simulink model "teste_motor_v10"  (R2025b)
settings: Solver=VariableStepAuto  StartTime=0.0  StopTime=10  RelTol=1e-3
undefined symbols (not defined in the file): fdesignblkfcn, gcbh, Kad, Kre
libraries: nesl_utility x26, fl_lib x25, simulink x19, dsparch4 x3, sdl_lib x2, simulink_extras x2, dspfdesign x1
(part 1 of 3)
CloseFcn:
  | try, close(h1_sdl_single_cylinder_engine), end
  | clear h1_sdl_single_cylinder_engine
  | 
  | clear simlog_sdl_single_cylinder_engine
  | clear logsout_sdl_single_cylinder_engine
settings Model: PacingRate=0.089000  Creator=The MathWorks, Inc.  LastModifiedBy=vclau
settings SolverCC: MaxZcPerStep=1.0
settings DataIOCC: SaveFormat=Array  SaveOutput=off  DSMLogging=off  SaveTime=off  ReturnWorkspaceOutputs=off  SignalLoggingName=logsout_sdl_single_cylinder_engine
settings DebuggingCC: AlgebraicLoopMsg=none  MaxConsecutiveZCsMsg=warning
settings ModelReferenceCC: EnableRefExpFcnMdlSchedulingChecks=on
settings RTWCC: GPUComputeCapability=3.5  DLArmComputeVersion=19.05
settings SimscapeCC: SimscapeLogType=all  SimscapeLogSimulationStatistics=on  SimscapeLogName=simlog_sdl_single_cylinder_engine  SimscapeLogLimitData=off

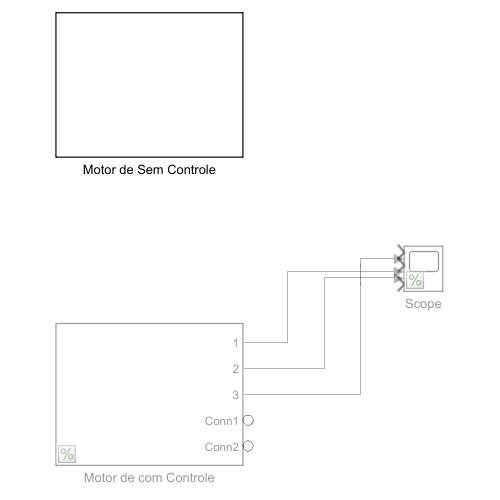
[thumbnail: Simulink's stored preview of the top-level diagram]
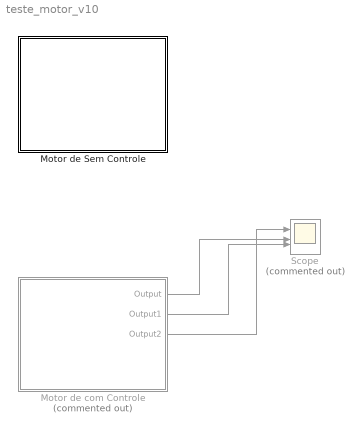
== system teste_motor_v10 ==
  Motor de Sem Controle : Subsystem
  Motor de com Controle : Subsystem  Commented=on
  Scope : Scope  Commented=on  NumInputPorts=6
      settings: ActiveDisplayYMinimum=-1  ActiveDisplayYMaximum=1
  wires:
  Motor de com Controle/1(Output) -> Scope/4
  Motor de com Controle/3(Output2) -> Scope/2
  Motor de com Controle/2(Output1) -> Scope/5

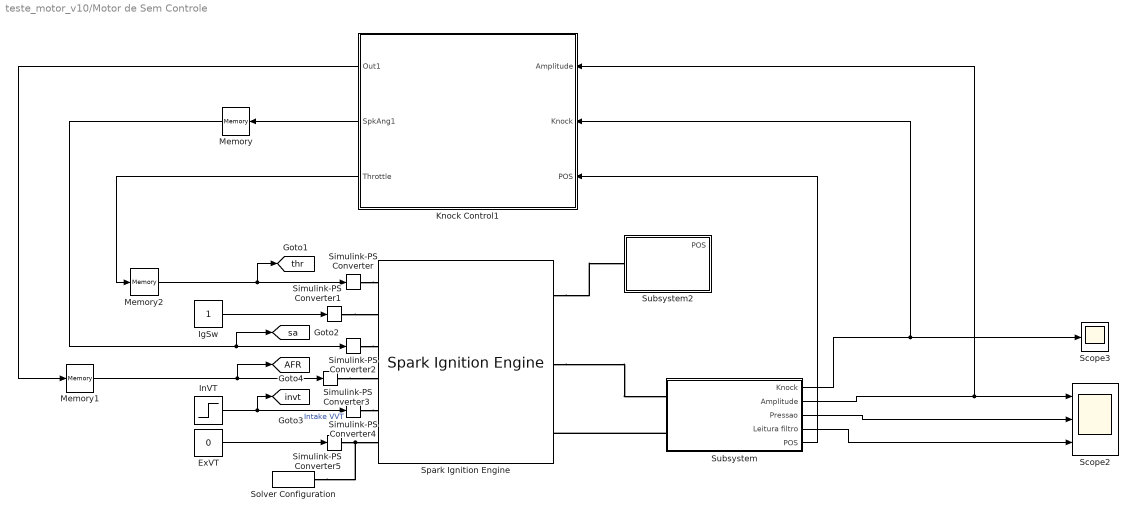
== system teste_motor_v10/Motor de Sem Controle ==
  ExVT : Constant  Value=0
  IgSw : Constant
  InVT : Step  Time=3  Before=30  After=0  SampleTime=0
  Knock Control1 : Subsystem
  Memory : Memory
  Memory1 : Memory  InitialCondition=14.7
  Memory2 : Memory
  Scope2 : Scope  NumInputPorts=3
      settings: ActiveDisplayYMinimum=-82.146412310849357  ActiveDisplayYMaximum=739.31771079764439  DataLoggingVariableName=ScopeData2
  Scope3 : Scope
      settings: ActiveDisplayYMinimum=0.61074348863970962  ActiveDisplayYMaximum=0.63050497432299946  DataLoggingVariableName=ScopeData3
  Simulink-PS Converter : nesl_utility/Simulink-PS Converter  PhysicalDomain=network_engine_domain  SubClassName=ps_input  LeftPortType=input  RightPortType=output  PseudoPeriodic=off  Frequencies=[]  NoiseDistribution=none  NoiseParameters=[]  Unit=1  AffineConversion=off  FilteringAndDerivatives=provide  SimscapeFilterOrder=1  InputFilterTimeConstant=0.001  UdotUserProvided=0
  Simulink-PS Converter1 : nesl_utility/Simulink-PS Converter  PhysicalDomain=network_engine_domain  SubClassName=ps_input  LeftPortType=input  RightPortType=output  PseudoPeriodic=off  Frequencies=[]  NoiseDistribution=none  NoiseParameters=[]  Unit=1  AffineConversion=off  FilteringAndDerivatives=provide  SimscapeFilterOrder=1  InputFilterTimeConstant=0.001  UdotUserProvided=0
  Simulink-PS Converter2 : nesl_utility/Simulink-PS Converter  PhysicalDomain=network_engine_domain  SubClassName=ps_input  LeftPortType=input  RightPortType=output  PseudoPeriodic=off  Frequencies=[]  NoiseDistribution=none  NoiseParameters=[]  Unit=deg  AffineConversion=off  FilteringAndDerivatives=provide  SimscapeFilterOrder=1  InputFilterTimeConstant=0.001  UdotUserProvided=0
  Simulink-PS Converter3 : nesl_utility/Simulink-PS Converter  PhysicalDomain=network_engine_domain  SubClassName=ps_input  LeftPortType=input  RightPortType=output  PseudoPeriodic=off  Frequencies=[]  NoiseDistribution=none  NoiseParameters=[]  Unit=1  AffineConversion=off  FilteringAndDerivatives=provide  SimscapeFilterOrder=1  InputFilterTimeConstant=0.001  UdotUserProvided=0
  Simulink-PS Converter4 : nesl_utility/Simulink-PS Converter  PhysicalDomain=network_engine_domain  SubClassName=ps_input  LeftPortType=input  RightPortType=output  PseudoPeriodic=off  Frequencies=[]  NoiseDistribution=none  NoiseParameters=[]  Unit=deg  AffineConversion=off  FilteringAndDerivatives=provide  SimscapeFilterOrder=1  InputFilterTimeConstant=0.001  UdotUserProvided=0
  Simulink-PS Converter5 : nesl_utility/Simulink-PS Converter  PhysicalDomain=network_engine_domain  SubClassName=ps_input  LeftPortType=input  RightPortType=output  PseudoPeriodic=off  Frequencies=[]  NoiseDistribution=none  NoiseParameters=[]  Unit=deg  AffineConversion=off  FilteringAndDerivatives=provide  SimscapeFilterOrder=1  InputFilterTimeConstant=0.001  UdotUserProvided=0
  Solver Configuration : nesl_utility/Solver Configuration  PhysicalDomain=network_engine_domain  SubClassName=solver  LeftPortType=input  RightPortType=generic  Tones=[]  Harmonics=[]  SimulateNoise=off  Profile=off  UseLocalSampling=off  EnableSwitchedLinearOptims=on  FrequencyDomain=off  UseCCode=off  RelTol=0.001  AbsTol=0.001  MinStep=1e-09  ToWorkspace=off  RevertToSquareIcSolve=off  NumHomotopyIterations=100  PhasorMode=off  PhasorModeNumHarmonics=1  ConsistencySolver=NEWTON_FTOL  IndexReductionMethod=DerivativeReplacement  DoDC=off  ResidualTolerance=1e-09  ConsistencyTolSource=GLOBAL  ConsistencyAbsTol=0.001  ConsistencyRelTol=0.001  ConsistencyTolFactor=0.001  UseLocalSolver=off  LocalSolverChoice=NE_BACKWARD_EULER_ADVANCER  ResolveIndetEquations=on  FunctionEvalNumThread=1  LocalSolverSampleTime=0.001  DoFixedCost=off  MaxNonlinIter=3  MaxModeIter=2  ComputeImpulses=off  ImpulseIterations=2  LinearAlgebra=auto  LinearAlgebraNumThread=0  EquationFormulation=NE_TIME_EF  DelaysMemoryBudget=1024  AutomaticFiltering=on  FilteringTimeConstant=0.001  PartitionStorageMethod=AS_NEEDED  PartitionMemoryBudget=1024  PartitionMethod=ROBUST  MultibodyUseLocalSolver=off  MultibodyLocalSolverChoice=ODE1  MultibodyLocalSolverSampleTime=0.001
  Spark Ignition Engine : sdl_lib/Engines & Motors/Spark Ignition Engine  numCyls=sdl.enum.engineNumCylinders.One  twoCylSADiff=270 deg  L4FiringOrder=sdl.enum.engineFiringOrderFourCylinders.L4_1342  bore=72 mm  stroke=61 mm  conrod=97 mm  CR=11.3  P_amb=101.325 kPa  T_amb=298.15 K  rho_air=1.225 mg/cm^3  R_air=288.1965 J/(K*kg)  UseAirIntake=simscape.enum.onoff.on  c_thr=0.05 s  thr_rest=3 deg  D_plate=5 cm  S_leak=1 cm^2  V_im=500 cm^3  Cd_in=0.9  IVO_0=5 deg  IVC_0=60 deg  EVO_0=60 deg  EVC_0=5 deg  UseInVVT=simscape.enum.onoff.on  UseExVVT=simscape.enum.onoff.on  q_LHV=44.3 MJ/kg  InputAFR=simscape.enum.onoff.on  AFR_const=14.6  InputInjPw=simscape.enum.onoff.off  Sinj=6.5 mg/ms  SparkInputType=sdl.enum.engineSparkInputType.Angle  SA_const=20 deg  comb_bd=50 deg  dt_Pcyl_slow_decay=60 s  dt_Tcyl_slow_decay=600 s  dt_exh_decay=5 ms  InputBackPressure=simscape.enum.onoff.off  dP_exh=50 kPa  dw_exh=6000 rpm  UseExhaustThermal=simscape.enum.onoff.on  S_exh=1 m^2  M_exh=5 kg  C_exh=100 J/(K*kg)  k_gas=10 s  h_convection=100 W/(K*m^2)  k_radiation=0.3  SB=5.7e-8 W/(K^4*m^2)  Pim_0=101.325 kPa  ca0=0 deg  w0=1000 rpm  EngSpdSimLimit=10000 rpm  OutputTorqueAvr=simscape.enum.onoff.off  OutputSpeedAvr=simscape.enum.onoff.off  OutputCrkpos=simscape.enum.onoff.on  OutputPim=simscape.enum.onoff.off  OutputAirMassFlow=simscape.enum.onoff.off  OutputFuelMassFlow=simscape.enum.onoff.off  OutputAFR=false  OutputVcyl=false  OutputPcyl=simscape.enum.onoff.on  OutputTcyl=simscape.enum.onoff.off  OutputTexh=simscape.enum.onoff.off
      settings: AttributesFormatString=%<w0> [%<w0_unit>]  InternalSimscapePortConfiguration="{\"Bottom\":[],\"Left\":[{\"id\":\"thr_cmd\",\"label\":\"Thr\",\"type\":\"input\"},{\"id\":\"IGSW\",\"label\":\"IgSw\",\"type\":\"input\"},{\"id\":\"sa\",\"label\":\"SA\",\"type\":\"input\"},{\"id\":\"afr_in\",\"label\":\"AfrCmd\",\"type\":\"input\"},{\"id\":\"dIV\",\"label\":\"InVT\",\"type\":\"input\"},{\"id\":\"dEV\",\"label\":\"ExVT\",\"type\":\"input\"}],\"Right\":[{\"id\":\"F\",\"label\":\"F\",\"type\":\"foundation.mechanical.rotational.rotational\"},{\"id\":\"crkpos\",\"label\":\"crkpos\",\"type\":\"output\"},{\"id\":\"P_out\",\"label\":\"Pcyl\",\"type\":\"output\"}],\"Top\":[]}"
  Subsystem : Subsystem
  Subsystem2 : Subsystem
  tag scope: AFR=global, invt=global, sa=global, thr=global
  wires:
  IgSw/1 -> Simulink-PS Converter1/1
  ExVT/1 -> Simulink-PS Converter5/1
  InVT/1 -> [invt], Simulink-PS Converter4/1  "Intake VVT"
  Subsystem/1(Knock) -> Knock Control1/2(Knock), Scope3/1
  Subsystem/2(Amplitude) -> Knock Control1/1(Amplitude), Scope2/1
  Subsystem/3(Pressao) -> Scope2/2
  Subsystem/4(Leitura filtro) -> Scope2/3
  Subsystem/5(POS) -> Knock Control1/3(POS)
  Memory/1 -> [sa], Simulink-PS Converter2/1
  Knock Control1/1(Out1) -> Memory1/1
  Memory1/1 -> [AFR], Simulink-PS Converter3/1
  Knock Control1/2(SpkAng1) -> Memory/1
  Knock Control1/3(Throttle) -> Memory2/1
  Memory2/1 -> [thr], Simulink-PS Converter/1
  connections:
  Simulink-PS Converter1/RConn1 -- Spark Ignition Engine/LConn2
  Simulink-PS Converter4/RConn1 -- Spark Ignition Engine/LConn5
  Simulink-PS Converter3/RConn1 -- Spark Ignition Engine/LConn4
  Simulink-PS Converter2/RConn1 -- Spark Ignition Engine/LConn3
  Simulink-PS Converter/RConn1 -- Spark Ignition Engine/LConn1
  Simulink-PS Converter5/RConn1 -- Solver Configuration/RConn1 -- Spark Ignition Engine/LConn6
  Spark Ignition Engine/RConn2 -- Subsystem/LConn1
  Subsystem/LConn2 -- Spark Ignition Engine/RConn3
  Spark Ignition Engine/RConn1 -- Subsystem2/LConn1

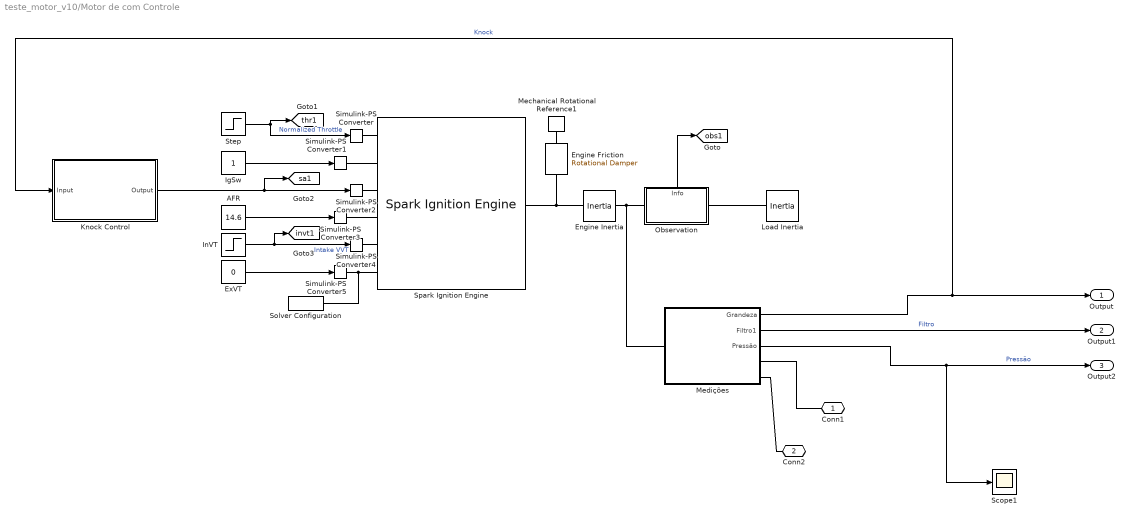
== system teste_motor_v10/Motor de com Controle ==
  AFR : Constant  Value=14.6
  Engine Friction : fl_lib/Mechanical/Rotational Elements/Rotational Damper  D=0.01 N*m/rpm  w_specify=off  w_priority=None  w=0 rad/s  w_nominal_specify=off  w_nominal_value=1  w_nominal_unit=rad/s  t_specify=off  t_priority=None  t=0 N*m  t_nominal_specify=off  t_nominal_value=1  t_nominal_unit=N*m
      settings: AttributesFormatString=%<D> [%<D_unit>]
  Engine Inertia : fl_lib/Mechanical/Rotational Elements/Inertia  inertia=0.01 kg*m^2  num_ports=foundation.enum.numPorts2.two  w_specify=on  w_priority=High  w=1000 rpm  w_nominal_specify=off  w_nominal_value=1  w_nominal_unit=rad/s  t_specify=off  t_priority=None  t=0 N*m  t_nominal_specify=off  t_nominal_value=1  t_nominal_unit=N*m
      settings: InternalSimscapePortConfiguration="{\"Bottom\":[],\"Left\":[{\"id\":\"I\",\"label\":\"\",\"type\":\"foundation.mechanical.rotational.rotational\"}],\"Right\":[{\"id\":\"J\",\"label\":\"\",\"type\":\"foundation.mechanical.rotational.rotational\"}],\"Top\":[]}"
      settings: AttributesFormatString=|
      | Initial: %<w> [%<w_unit>]
      | %<inertia> [%<inertia_unit>]
  ExVT : Constant  Value=0
  IgSw : Constant
  InVT : Step  Time=3  Before=30  After=0  SampleTime=0
  Knock Control : Subsystem
  Load Inertia : fl_lib/Mechanical/Rotational Elements/Inertia  inertia=10*0.1^2 kg*m^2  num_ports=foundation.enum.numPorts2.one  w_specify=on  w_priority=None  w=0 rpm  w_nominal_specify=off  w_nominal_value=1  w_nominal_unit=rad/s  t_specify=off  t_priority=None  t=0 N*m  t_nominal_specify=off  t_nominal_value=1  t_nominal_unit=N*m
      settings: AttributesFormatString=|
      | Initial: %<w> [%<w_unit>]
      | %<inertia> [%<inertia_unit>]
  Mechanical Rotational Reference1 : fl_lib/Mechanical/Rotational Elements/Mechanical Rotational Reference
  Medições : Subsystem
  Observation : Subsystem
      settings: PortSchema="{\"entries\":[{\"content\":{\"sides\":[{\"content\":{\"connectorIds\":[\"LConn1\"]},\"type\":\"ConnectorPlacement.EquallySpacedRectSide\",\"uuid\":\"410be9a6-c4e5-432d-8066-24e0f4965a53\"},{\"content\":{\"connectorIds\":[\"RConn1\"],\"side\":\"RIGHT\"},\"type\":\"ConnectorPlacement.EquallySpacedRectSide\",\"uuid\":\"7b59f0c0-a218-4635-982c-3ab19ae33344\"},{\"content\":{\"connectorIds\":[\"Out1\"],\"side\":\"TOP\"},\"type\":\"ConnectorPlacement.EquallySpacedRectSide\",\"uuid\":\"569b4327-99bc-47a9-a8b7-c1caa6dee46d\"}]},\"type\":\"ConnectorPlacement.EquallySpacedConnector\",\"uuid\":\"611a8619-a64a-4be7-a61a-aa8fabb87e61\"}],\"packageUris\":[\"http://schema.mathworks.com/mf0/Connector/R2020b\"],\"version\":\"1.0\"}"
  Scope1 : Scope
      settings: ActiveDisplayYMinimum=101298.89151  ActiveDisplayYMaximum=101559.9764  DataLoggingVariableName=ScopeData3
  Simulink-PS Converter : nesl_utility/Simulink-PS Converter  PhysicalDomain=network_engine_domain  SubClassName=ps_input  LeftPortType=input  RightPortType=output  PseudoPeriodic=off  Frequencies=[]  NoiseDistribution=none  NoiseParameters=[]  Unit=1  AffineConversion=off  FilteringAndDerivatives=provide  SimscapeFilterOrder=1  InputFilterTimeConstant=0.001  UdotUserProvided=0
  Simulink-PS Converter1 : nesl_utility/Simulink-PS Converter  PhysicalDomain=network_engine_domain  SubClassName=ps_input  LeftPortType=input  RightPortType=output  PseudoPeriodic=off  Frequencies=[]  NoiseDistribution=none  NoiseParameters=[]  Unit=1  AffineConversion=off  FilteringAndDerivatives=provide  SimscapeFilterOrder=1  InputFilterTimeConstant=0.001  UdotUserProvided=0
  Simulink-PS Converter2 : nesl_utility/Simulink-PS Converter  PhysicalDomain=network_engine_domain  SubClassName=ps_input  LeftPortType=input  RightPortType=output  PseudoPeriodic=off  Frequencies=[]  NoiseDistribution=none  NoiseParameters=[]  Unit=deg  AffineConversion=off  FilteringAndDerivatives=provide  SimscapeFilterOrder=1  InputFilterTimeConstant=0.001  UdotUserProvided=0
  Simulink-PS Converter3 : nesl_utility/Simulink-PS Converter  PhysicalDomain=network_engine_domain  SubClassName=ps_input  LeftPortType=input  RightPortType=output  PseudoPeriodic=off  Frequencies=[]  NoiseDistribution=none  NoiseParameters=[]  Unit=1  AffineConversion=off  FilteringAndDerivatives=provide  SimscapeFilterOrder=1  InputFilterTimeConstant=0.001  UdotUserProvided=0
  Simulink-PS Converter4 : nesl_utility/Simulink-PS Converter  PhysicalDomain=network_engine_domain  SubClassName=ps_input  LeftPortType=input  RightPortType=output  PseudoPeriodic=off  Frequencies=[]  NoiseDistribution=none  NoiseParameters=[]  Unit=deg  AffineConversion=off  FilteringAndDerivatives=provide  SimscapeFilterOrder=1  InputFilterTimeConstant=0.001  UdotUserProvided=0
  Simulink-PS Converter5 : nesl_utility/Simulink-PS Converter  PhysicalDomain=network_engine_domain  SubClassName=ps_input  LeftPortType=input  RightPortType=output  PseudoPeriodic=off  Frequencies=[]  NoiseDistribution=none  NoiseParameters=[]  Unit=deg  AffineConversion=off  FilteringAndDerivatives=provide  SimscapeFilterOrder=1  InputFilterTimeConstant=0.001  UdotUserProvided=0
  Solver Configuration : nesl_utility/Solver Configuration  PhysicalDomain=network_engine_domain  SubClassName=solver  LeftPortType=input  RightPortType=generic  Tones=[]  Harmonics=[]  SimulateNoise=off  Profile=off  UseLocalSampling=off  EnableSwitchedLinearOptims=on  FrequencyDomain=off  UseCCode=off  RelTol=0.001  AbsTol=0.001  MinStep=1e-09  ToWorkspace=off  RevertToSquareIcSolve=off  NumHomotopyIterations=100  PhasorMode=off  PhasorModeNumHarmonics=1  ConsistencySolver=NEWTON_FTOL  IndexReductionMethod=DerivativeReplacement  DoDC=off  ResidualTolerance=1e-09  ConsistencyTolSource=GLOBAL  ConsistencyAbsTol=0.001  ConsistencyRelTol=0.001  ConsistencyTolFactor=0.001  UseLocalSolver=off  LocalSolverChoice=NE_BACKWARD_EULER_ADVANCER  ResolveIndetEquations=on  FunctionEvalNumThread=1  LocalSolverSampleTime=0.001  DoFixedCost=off  MaxNonlinIter=3  MaxModeIter=2  ComputeImpulses=off  ImpulseIterations=2  LinearAlgebra=auto  LinearAlgebraNumThread=0  EquationFormulation=NE_TIME_EF  DelaysMemoryBudget=1024  AutomaticFiltering=on  FilteringTimeConstant=0.001  PartitionStorageMethod=AS_NEEDED  PartitionMemoryBudget=1024  PartitionMethod=ROBUST  MultibodyUseLocalSolver=off  MultibodyLocalSolverChoice=ODE1  MultibodyLocalSolverSampleTime=0.001
  Spark Ignition Engine : sdl_lib/Engines & Motors/Spark Ignition Engine  numCyls=sdl.enum.engineNumCylinders.One  twoCylSADiff=270 deg  L4FiringOrder=sdl.enum.engineFiringOrderFourCylinders.L4_1342  bore=72 mm  stroke=61 mm  conrod=97 mm  CR=11.3  P_amb=101.325 kPa  T_amb=298.15 K  rho_air=1.225 mg/cm^3  R_air=288.1965 J/(K*kg)  UseAirIntake=simscape.enum.onoff.on  c_thr=0.05 s  thr_rest=3 deg  D_plate=5 cm  S_leak=1 cm^2  V_im=500 cm^3  Cd_in=0.9  IVO_0=5 deg  IVC_0=60 deg  EVO_0=60 deg  EVC_0=5 deg  UseInVVT=simscape.enum.onoff.on  UseExVVT=simscape.enum.onoff.on  q_LHV=44.3 MJ/kg  InputAFR=simscape.enum.onoff.on  AFR_const=14.6  InputInjPw=simscape.enum.onoff.off  Sinj=6.5 mg/ms  SparkInputType=sdl.enum.engineSparkInputType.Angle  SA_const=20 deg  comb_bd=50 deg  dt_Pcyl_slow_decay=60 s  dt_Tcyl_slow_decay=600 s  dt_exh_decay=5 ms  InputBackPressure=simscape.enum.onoff.off  dP_exh=50 kPa  dw_exh=6000 rpm  UseExhaustThermal=simscape.enum.onoff.on  S_exh=1 m^2  M_exh=5 kg  C_exh=100 J/(K*kg)  k_gas=10 s  h_convection=100 W/(K*m^2)  k_radiation=0.3  SB=5.7e-8 W/(K^4*m^2)  Pim_0=101.325 kPa  ca0=0 deg  w0=1000 rpm  EngSpdSimLimit=10000 rpm  OutputTorqueAvr=simscape.enum.onoff.off  OutputSpeedAvr=simscape.enum.onoff.off  OutputCrkpos=simscape.enum.onoff.off  OutputPim=simscape.enum.onoff.off  OutputAirMassFlow=simscape.enum.onoff.off  OutputFuelMassFlow=simscape.enum.onoff.off  OutputAFR=simscape.enum.onoff.off  OutputVcyl=simscape.enum.onoff.off  OutputPcyl=simscape.enum.onoff.off  OutputTcyl=simscape.enum.onoff.off  OutputTexh=simscape.enum.onoff.off
      settings: AttributesFormatString=%<w0> [%<w0_unit>]  InternalSimscapePortConfiguration="{\"Bottom\":[],\"Left\":[{\"id\":\"thr_cmd\",\"label\":\"Thr\",\"type\":\"input\"},{\"id\":\"IGSW\",\"label\":\"IgSw\",\"type\":\"input\"},{\"id\":\"sa\",\"label\":\"SA\",\"type\":\"input\"},{\"id\":\"afr_in\",\"label\":\"AfrCmd\",\"type\":\"input\"},{\"id\":\"dIV\",\"label\":\"InVT\",\"type\":\"input\"},{\"id\":\"dEV\",\"label\":\"ExVT\",\"type\":\"input\"}],\"Right\":[{\"id\":\"F\",\"label\":\"F\",\"type\":\"foundation.mechanical.rotational.rotational\"}],\"Top\":[]}"
  Step : Step  Time=15  Before=0.2  SampleTime=0
  Conn1 : PMIOPort  Side=Right
  Conn2 : PMIOPort  Port=2  Side=Right
  Output : Outport
  Output1 : Outport  Port=2
  Output2 : Outport  Port=3
  tag scope: invt1=global, obs1=global, sa1=global, thr1=global
  wires:
  IgSw/1 -> Simulink-PS Converter1/1
  Medições/2(Filtro1) -> Output1/1  "Filtro"
  AFR/1 -> Simulink-PS Converter3/1
  Step/1 -> Simulink-PS Converter/1, [thr1]  "Normalized Throttle"
  Observation/1(Info) -> [obs1]
  Medições/1(Grandeza) -> Output/1, Knock Control/1(Input)  "Knock"
  Knock Control/1(Output) -> [sa1], Simulink-PS Converter2/1
  ExVT/1 -> Simulink-PS Converter5/1
  Medições/3(Pressão) -> Output2/1, Scope1/1  "Pressão"
  InVT/1 -> [invt1], Simulink-PS Converter4/1  "Intake VVT"
  connections:
  Medições/RConn1 -- Conn1/RConn1
  Spark Ignition Engine/RConn1 -- Engine Friction/LConn1 -- Engine Inertia/RConn1
  Simulink-PS Converter1/RConn1 -- Spark Ignition Engine/LConn2
  Mechanical Rotational Reference1/LConn1 -- Engine Friction/RConn1
  Simulink-PS Converter4/RConn1 -- Spark Ignition Engine/LConn5
  Observation/RConn1 -- Load Inertia/LConn1
  Simulink-PS Converter3/RConn1 -- Spark Ignition Engine/LConn4
  Simulink-PS Converter2/RConn1 -- Spark Ignition Engine/LConn3
  Simulink-PS Converter/RConn1 -- Spark Ignition Engine/LConn1
  Engine Inertia/LConn1 -- Medições/LConn1 -- Observation/LConn1
  Simulink-PS Converter5/RConn1 -- Solver Configuration/RConn1 -- Spark Ignition Engine/LConn6
  Medições/RConn2 -- Conn2/RConn1

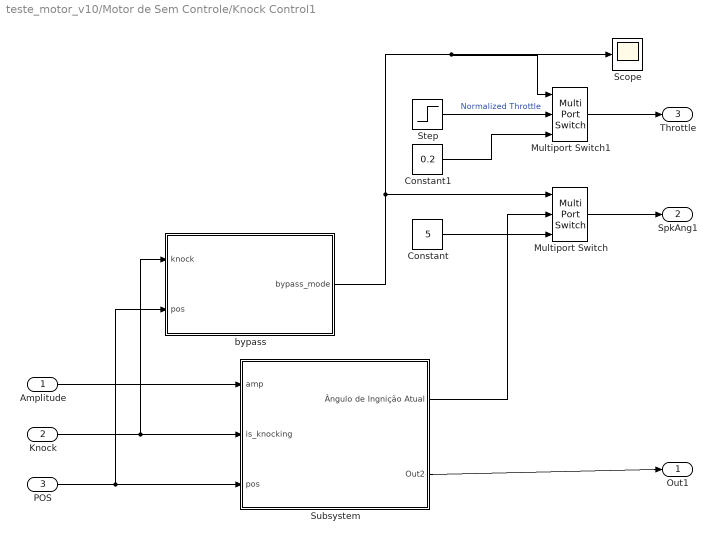
== system teste_motor_v10/Motor de Sem Controle/Knock Control1 ==
  Amplitude : Inport
  Knock : Inport  Port=2
  POS : Inport  Port=3
  Constant : Constant  Value=5
  Constant1 : Constant  Value=0.2
  Multiport Switch : MultiPortSwitch  Inputs=2  SaturateOnIntegerOverflow=off  InputSameDT=off
  Multiport Switch1 : MultiPortSwitch  Inputs=2  SaturateOnIntegerOverflow=off  InputSameDT=off
  Scope : Scope
      settings: ActiveDisplayYMinimum=0.875  ActiveDisplayYMaximum=2.125  DataLoggingVariableName=ScopeData12
  Step : Step  Before=0.2  SampleTime=0
  Subsystem : Subsystem
  bypass : MATLAB Function  TreatAsAtomicUnit=on
  Out1 : Outport
  SpkAng1 : Outport  Port=2
  Throttle : Outport  Port=3
  wires:
  Amplitude/1 -> Subsystem/1(amp)
  Knock/1 -> bypass/1(knock), Subsystem/2(is_knocking)
  POS/1 -> bypass/2(pos), Subsystem/3(pos)
  Subsystem/2(Out2) -> Out1/1
  Subsystem/1(Ângulo de Ingnição Atual) -> Multiport Switch/2
  Multiport Switch/1 -> SpkAng1/1
  Multiport Switch1/1 -> Throttle/1
  Step/1 -> Multiport Switch1/2  "Normalized Throttle"
  bypass/1(bypass_mode) -> Scope/1, Multiport Switch1/1, Multiport Switch/1
  Constant/1 -> Multiport Switch/3
  Constant1/1 -> Multiport Switch1/3

== system teste_motor_v10/Motor de Sem Controle/Subsystem ==
  Filtro : Subsystem
  Leituras : Subsystem
  Threshold e Sensor : Subsystem
  Crank Angle : PMIOPort  Side=Left
  Pressão : PMIOPort  Port=2  Side=Left
  Knock : Outport
  Amplitude : Outport  Port=2
  Pressao : Outport  Port=3
  Leitura filtro : Outport  Port=4
  POS : Outport  Port=5
  wires:
  Leituras/1(Pressão com Knock) -> Pressao/1, Filtro/1(Pressão com Knock)
  Threshold e Sensor/1(Knock) -> Knock/1
  Filtro/2(Filtro) -> Leitura filtro/1
  Threshold e Sensor/2(Amplitude) -> Amplitude/1
  Filtro/1(Sinal filtrado) -> Threshold e Sensor/1(Sinal filtrado)
  Leituras/2(CrkAng) -> POS/1
  connections:
  Crank Angle/RConn1 -- Leituras/LConn1
  Leituras/LConn2 -- Pressão/RConn1

== system teste_motor_v10/Motor de Sem Controle/Subsystem2 ==
  Engine Friction : fl_lib/Mechanical/Rotational Elements/Rotational Damper  D=0.01 N*m/rpm  w_specify=off  w_priority=None  w=0 rad/s  w_nominal_specify=off  w_nominal_value=1  w_nominal_unit=rad/s  t_specify=off  t_priority=None  t=0 N*m  t_nominal_specify=off  t_nominal_value=1  t_nominal_unit=N*m
      settings: AttributesFormatString=%<D> [%<D_unit>]
  Engine Inertia : fl_lib/Mechanical/Rotational Elements/Inertia  inertia=0.01 kg*m^2  num_ports=foundation.enum.numPorts2.two  w_specify=on  w_priority=High  w=1000 rpm  w_nominal_specify=off  w_nominal_value=1  w_nominal_unit=rad/s  t_specify=off  t_priority=None  t=0 N*m  t_nominal_specify=off  t_nominal_value=1  t_nominal_unit=N*m
      settings: InternalSimscapePortConfiguration="{\"Bottom\":[],\"Left\":[{\"id\":\"I\",\"label\":\"\",\"type\":\"foundation.mechanical.rotational.rotational\"}],\"Right\":[{\"id\":\"J\",\"label\":\"\",\"type\":\"foundation.mechanical.rotational.rotational\"}],\"Top\":[]}"
      settings: AttributesFormatString=|
      | Initial: %<w> [%<w_unit>]
      | %<inertia> [%<inertia_unit>]
  Load Inertia : fl_lib/Mechanical/Rotational Elements/Inertia  inertia=10*0.1^2 kg*m^2  num_ports=foundation.enum.numPorts2.one  w_specify=on  w_priority=None  w=0 rpm  w_nominal_specify=off  w_nominal_value=1  w_nominal_unit=rad/s  t_specify=off  t_priority=None  t=0 N*m  t_nominal_specify=off  t_nominal_value=1  t_nominal_unit=N*m
      settings: AttributesFormatString=|
      | Initial: %<w> [%<w_unit>]
      | %<inertia> [%<inertia_unit>]
  Mechanical Rotational Reference1 : fl_lib/Mechanical/Rotational Elements/Mechanical Rotational Reference
  Observation : Subsystem
      settings: PortSchema="{\"entries\":[{\"content\":{\"sides\":[{\"content\":{\"connectorIds\":[\"LConn1\"]},\"type\":\"ConnectorPlacement.EquallySpacedRectSide\",\"uuid\":\"410be9a6-c4e5-432d-8066-24e0f4965a53\"},{\"content\":{\"connectorIds\":[\"RConn1\"],\"side\":\"RIGHT\"},\"type\":\"ConnectorPlacement.EquallySpacedRectSide\",\"uuid\":\"7b59f0c0-a218-4635-982c-3ab19ae33344\"},{\"content\":{\"connectorIds\":[\"Out1\"],\"side\":\"TOP\"},\"type\":\"ConnectorPlacement.EquallySpacedRectSide\",\"uuid\":\"569b4327-99bc-47a9-a8b7-c1caa6dee46d\"}]},\"type\":\"ConnectorPlacement.EquallySpacedConnector\",\"uuid\":\"611a8619-a64a-4be7-a61a-aa8fabb87e61\"}],\"packageUris\":[\"http://schema.mathworks.com/mf0/Connector/R2020b\"],\"version\":\"1.0\"}"
  Subsystem1 : Subsystem
  Conn1 : PMIOPort  Side=Left
  Conn2 : PMIOPort  Port=2  Side=Right
  Conn3 : PMIOPort  Port=3  Side=Right
  POS : Outport
  tag scope: obs=global
  wires:
  Subsystem1/1(POS) -> POS/1
  Observation/1(Info) -> [obs]
  connections:
  Engine Friction/LConn1 -- Conn1/RConn1 -- Engine Inertia/RConn1
  Mechanical Rotational Reference1/LConn1 -- Engine Friction/RConn1
  Engine Inertia/LConn1 -- Subsystem1/LConn1 -- Observation/LConn1
  Subsystem1/RConn1 -- Conn2/RConn1
  Observation/RConn1 -- Load Inertia/LConn1
  Subsystem1/RConn2 -- Conn3/RConn1

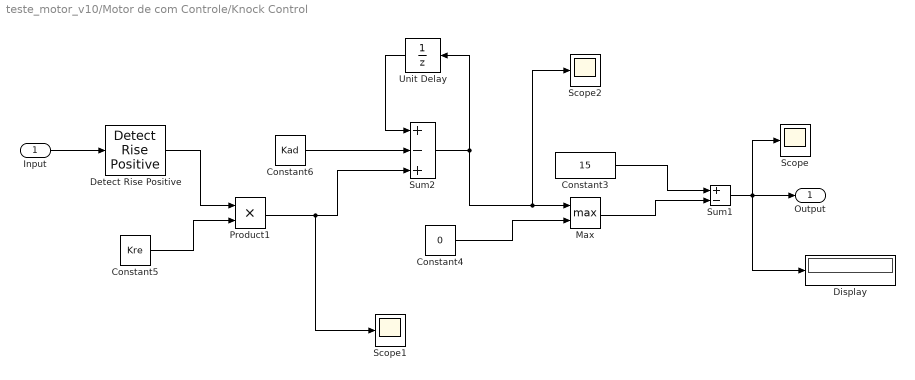
== system teste_motor_v10/Motor de com Controle/Knock Control ==
  Input : Inport
  Constant3 : Constant  Value=15
  Constant4 : Constant  Value=0
  Constant5 : Constant  Value=Kre
  Constant6 : Constant  Value=Kad
  Detect Rise Positive : simulink/Logic and Bit Operations/Detect Rise Positive  vinit=0  OutDataTypeStr=boolean
  Display : Display
  Max : MinMax  Function=max  Inputs=2
  Product1 : Product
  Scope : Scope
      settings: ActiveDisplayYMinimum=11.265  ActiveDisplayYMaximum=15.415
  Scope1 : Scope
      settings: ActiveDisplayYMinimum=-0.625  ActiveDisplayYMaximum=5.625
  Scope2 : Scope
      settings: ActiveDisplayYMinimum=-23.7475  ActiveDisplayYMaximum=6.3275  DataLoggingVariableName=ScopeData2
  Sum1 : Sum  Inputs=+-
  Sum2 : Sum  Inputs=+-+
  Unit Delay : UnitDelay  SampleTime=-1  HasFrameUpgradeWarning=on
  Output : Outport
  wires:
  Constant3/1 -> Sum1/1
  Max/1 -> Sum1/2
  Sum2/1 -> Unit Delay/1, Scope2/1, Max/1
  Product1/1 -> Scope1/1, Sum2/3
  Constant4/1 -> Max/2
  Constant6/1 -> Sum2/2
  Constant5/1 -> Product1/2
  Sum1/1 -> Display/1, Scope/1, Output/1
  Unit Delay/1 -> Sum2/1
  Detect Rise Positive/1 -> Product1/1
  Input/1 -> Detect Rise Positive/1

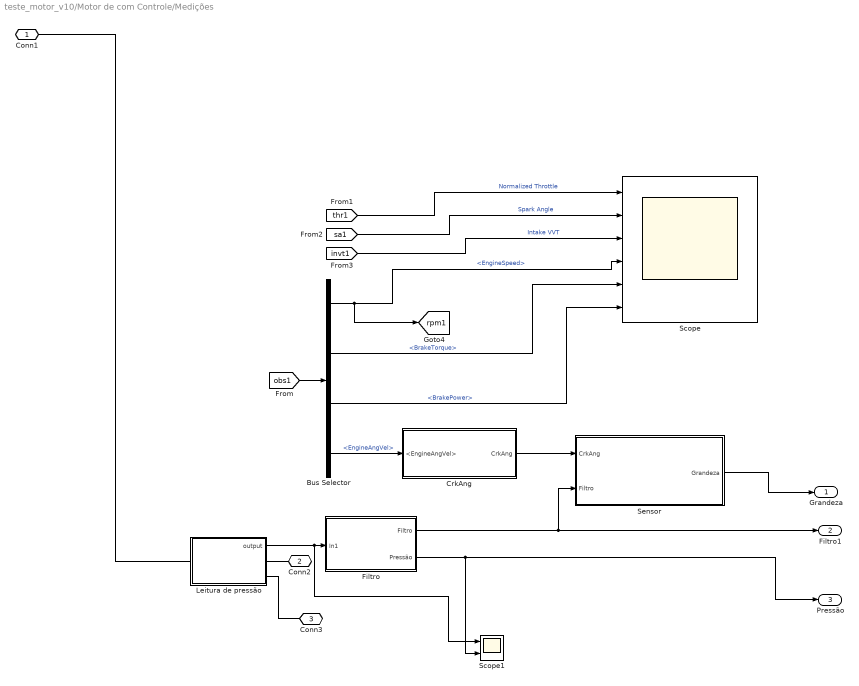
== system teste_motor_v10/Motor de com Controle/Medições ==
  Bus Selector : BusSelector  OutputSignals=EngineSpeed,BrakeTorque,BrakePower,EngineAngVel
  CrkAng : Subsystem
  Filtro : Subsystem
  Leitura de pressão : Subsystem
  Scope : Scope  NumInputPorts=6
      settings: ActiveDisplayYMinimum=0.1  ActiveDisplayYMaximum=1.1
  Scope1 : Scope  NumInputPorts=2
      settings: ActiveDisplayYMinimum=94814.33534  ActiveDisplayYMaximum=119364.22182  DataLoggingVariableName=ScopeData5
  Sensor : Subsystem
  Conn1 : PMIOPort  Side=Left
  Conn2 : PMIOPort  Port=2  Side=Right
  Conn3 : PMIOPort  Port=3  Side=Right
  Grandeza : Outport
  Filtro1 : Outport  Port=2
  Pressão : Outport  Port=3
  tag scope: rpm1=global
  wires:
  [invt1] -> Scope/3  "Intake VVT"
  CrkAng/1(CrkAng) -> Sensor/1(CrkAng)
  Filtro/1(Filtro) -> Filtro1/1, Sensor/2(Filtro)
  [obs1] -> Bus Selector/1
  Bus Selector/4 -> CrkAng/1(<EngineAngVel>)  "<EngineAngVel>"
  Leitura de pressão/1(output) -> Scope1/1, Filtro/1(In1)
  Bus Selector/2 -> Scope/5  "<BrakeTorque>"
  Bus Selector/3 -> Scope/6  "<BrakePower>"
  Bus Selector/1 -> [rpm1], Scope/4  "<EngineSpeed>"
  [sa1] -> Scope/2  "Spark Angle"
  [thr1] -> Scope/1  "Normalized Throttle"
  Filtro/2(Pressão) -> Scope1/2, Pressão/1
  Sensor/1(Grandeza) -> Grandeza/1
  connections:
  Leitura de pressão/RConn1 -- Conn2/RConn1
  Leitura de pressão/LConn1 -- Conn1/RConn1
  Leitura de pressão/RConn2 -- Conn3/RConn1

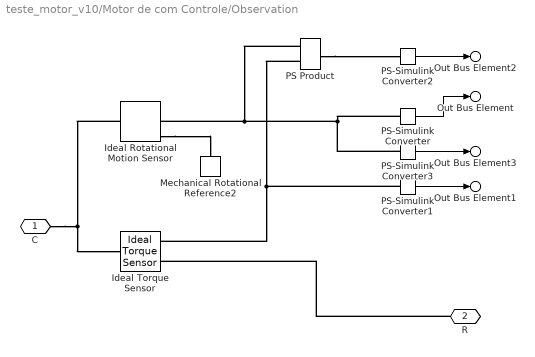
== system teste_motor_v10/Motor de com Controle/Observation ==
  Ideal Rotational Motion Sensor : fl_lib/Mechanical/Mechanical Sensors/Ideal Rotational Motion Sensor  reference=foundation.enum.MeasurementReference.difference  acceleration_port=false  velocity_port=true  position_port=true  wrap_angle=simscape.enum.onoff.off  offset=0 rad
  Ideal Torque Sensor : fl_lib/Mechanical/Mechanical Sensors/Ideal Torque Sensor
  Mechanical Rotational Reference2 : fl_lib/Mechanical/Rotational Elements/Mechanical Rotational Reference
  PS Product : fl_lib/Physical Signals/Functions/PS Product
  PS-Simulink Converter : nesl_utility/PS-Simulink Converter  PhysicalDomain=network_engine_domain  SubClassName=ps_output  LeftPortType=input  RightPortType=output  PseudoPeriodic=off  Frequencies=[]  VectorFormat=inherit  Unit=rpm  AffineConversion=off
  PS-Simulink Converter1 : nesl_utility/PS-Simulink Converter  PhysicalDomain=network_engine_domain  SubClassName=ps_output  LeftPortType=input  RightPortType=output  PseudoPeriodic=off  Frequencies=[]  VectorFormat=inherit  Unit=N*m  AffineConversion=off
  PS-Simulink Converter2 : nesl_utility/PS-Simulink Converter  PhysicalDomain=network_engine_domain  SubClassName=ps_output  LeftPortType=input  RightPortType=output  PseudoPeriodic=off  Frequencies=[]  VectorFormat=inherit  Unit=kW  AffineConversion=off
  PS-Simulink Converter3 : nesl_utility/PS-Simulink Converter  PhysicalDomain=network_engine_domain  SubClassName=ps_output  LeftPortType=input  RightPortType=output  PseudoPeriodic=off  Frequencies=[]  VectorFormat=inherit  Unit=rad/s  AffineConversion=off
  C : PMIOPort  Side=Left
  R : PMIOPort  Port=2  Side=Right
  Out Bus Element : Outport  PortName=Info  Element=EngineSpeed
      settings: AttributesFormatString=%<Unit>
  Out Bus Element1 : Outport  PortName=Info  Element=BrakeTorque
      settings: AttributesFormatString=%<Unit>
  Out Bus Element2 : Outport  PortName=Info  Element=BrakePower
      settings: AttributesFormatString=%<Unit>
  Out Bus Element3 : Outport  PortName=Info  Element=EngineAngVel
      settings: AttributesFormatString=%<Unit>
  wires:
  PS-Simulink Converter/1 -> Out Bus Element/1
  PS-Simulink Converter1/1 -> Out Bus Element1/1
  PS-Simulink Converter2/1 -> Out Bus Element2/1
  PS-Simulink Converter3/1 -> Out Bus Element3/1
  connections:
  Ideal Rotational Motion Sensor/RConn1 -- Mechanical Rotational Reference2/LConn1
  Ideal Rotational Motion Sensor/LConn1 -- C/RConn1 -- Ideal Torque Sensor/LConn1
  PS-Simulink Converter/LConn1 -- PS-Simulink Converter3/LConn1 -- PS Product/LConn1 -- Ideal Rotational Motion Sensor/RConn2
  PS-Simulink Converter1/LConn1 -- PS Product/LConn2 -- Ideal Torque Sensor/RConn2
  R/RConn1 -- Ideal Torque Sensor/RConn1
  PS Product/RConn1 -- PS-Simulink Converter2/LConn1

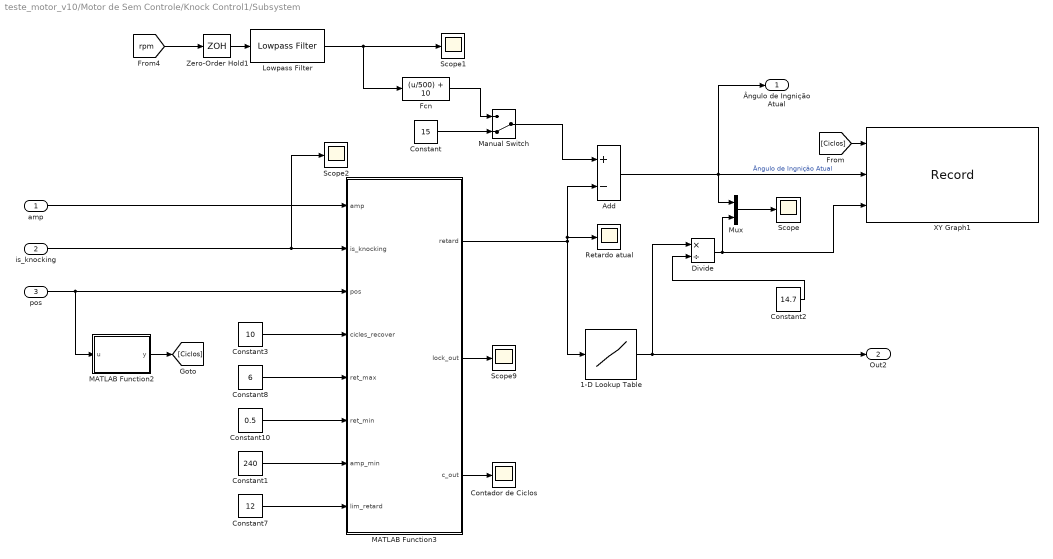
== system teste_motor_v10/Motor de Sem Controle/Knock Control1/Subsystem ==
  amp : Inport
  is_knocking : Inport  Port=2
  pos : Inport  Port=3
  1-D Lookup Table : Lookup_n-D  NumberOfTableDimensions=1  BreakpointsForDimension1=[0, 10, 12, 16]  Table=[14.7, 14.7, 11.76, 11.76]  InternalRulePriority=Speed  RndMeth=Simplest
  Add : Sum  Inputs=+-
  Constant : Constant  Value=15
  Constant1 : Constant  Value=240
  Constant10 : Constant  Value=0.5
  Constant2 : Constant  Value=14.7
  Constant3 : Constant  Value=10
  Constant7 : Constant  Value=12
  Constant8 : Constant  Value=6
  Contador de Ciclos : Scope
      settings: ActiveDisplayYMinimum=162.25  ActiveDisplayYMaximum=199.75  DataLoggingVariableName=ScopeData10
  Divide : Product  Inputs=*/
  Fcn : Fcn  Expr=(u/500) + 10
  Lowpass Filter : dspfdesign/Lowpass Filter  FilterType=FIR  DesignForMinimumOrder=on  FilterOrder=50  PassbandFrequency=5  StopbandFrequency=15  PassbandRipple=0.1  StopbandAttenuation=80  SampleRate=44100  SimulateUsing=Interpreted execution  roundingMode=Floor  coeffsDataTypeStr=fixdt(1,16)
  MATLAB Function2 : MATLAB Function  TreatAsAtomicUnit=on
  MATLAB Function3 : MATLAB Function  TreatAsAtomicUnit=on
  Manual Switch : ManualSwitch  CurrentSetting=0
  Mux : Mux  Inputs=2
  Retardo atual : Scope
      settings: ActiveDisplayYMinimum=-0.75  ActiveDisplayYMaximum=6.75  DataLoggingVariableName=ScopeData5
  Scope{,1..2,9} (4 alike) : Scope
      Scope settings: ActiveDisplayYMinimum=-0.74999999999999956  ActiveDisplayYMaximum=16.75  DataLoggingVariableName=ScopeData6
      Scope1 settings: ActiveDisplayYMinimum=-302.57065  ActiveDisplayYMaximum=2013.87294  DataLoggingVariableName=ScopeData4
      Scope2 settings: ActiveDisplayYMinimum=-0.12499999999999997  ActiveDisplayYMaximum=1.125  DataLoggingVariableName=ScopeData11
      Scope9 settings: ActiveDisplayYMinimum=-1  ActiveDisplayYMaximum=1  DataLoggingVariableName=ScopeData9
  XY Graph1 : Record  NumPorts=3.0  FileSettingsInternal="{\"entries\":[{\"content\":{\"excelSettings\":{\"content\":{},\"type\":\"Streamout.ExcelSettings\"},\"parquetSettings\":{\"content\":{},\"type\":\"Streamout.ParquetSettings\"}},\"type\":\"Streamout.FileSettingStorage\",\"uuid\":\"\"}],\"packageUris\":[\"http:\\/\\/schema.mathworks.com\\/mf0\\/streamout_blocks\\/R2020a\"],\"version\":\"1.0\"}"  FrameSettings=[0, 0, 0]  Layout=[1 1]  SignalsInternal="{\"entries\":[{\"content\":{\"signals\":[{\"content\":{\"blockPath\":[],\"dimensions\":[1],\"domain\":\"\",\"lineColor\":\"#22b573\",\"lineWidth\":2,\"port\":1,\"sid\":[\"\"],\"signalID\":1,\"signalName\":\"From\"},\"type\":\"RecordBlkView.Signal\",\"uuid\":\"\"},{\"content\":{\"blockPath\":[],\"dimensions\":[1],\"domain\":\"\",\"lineColor\":\"#0072bd\",\"lineWidth\":2,\"port\":2,\"sid\":[\"\"],\"signalID\":2,\"signalName\":\"Ângulo de Ingnição Atual\"},\"type\":\"RecordBlkView.Signal\",\"uuid\":\"\"},{\"content\":{\"blockPath\":[],\"dimensions\":[1],\"domain\":\"\",\"lineColor\":\"#d95319\",\"lineWidth\":2,\"port\":3,\"sid\":[\"\"],\"signalID\":3,\"signalName\":\"1-D Lookup\\nTable\"},\"type\":\"RecordBlkView.Signal\",\"uuid\":\"\"}]},\"type\":\"RecordBlkView.InputSignals\",\"uuid\":\"\"}],\"packageUris\":[\"http:\\/\\/schema.mathworks.com\\/mf0\\/streamout_blocks\\/R2020a\"],\"version\":\"1.0\"}"  VisualizationBindings="{\"xyplotplugin\":{\"info\":[{\"series\":[],\"subplotID\":1}]}}"  CompatibilityTag=XY
  Zero-Order Hold1 : ZeroOrderHold  SampleTime=-1
  Ângulo de Ingnição Atual : Outport
  Out2 : Outport  Port=2
  wires:
  Fcn/1 -> Manual Switch/1
  Lowpass Filter/1 -> Fcn/1, Scope1/1
  Add/1 -> Ângulo de Ingnição Atual/1, Mux/1, XY Graph1/2  "Ângulo de Ingnição Atual"
  Constant7/1 -> MATLAB Function3/8(lim_retard)
  Constant/1 -> Manual Switch/2
  is_knocking/1 -> Scope2/1, MATLAB Function3/2(is_knocking)
  Constant3/1 -> MATLAB Function3/4(cicles_recover)
  Constant1/1 -> MATLAB Function3/7(amp_min)
  pos/1 -> MATLAB Function3/3(pos), MATLAB Function2/1(u)
  Manual Switch/1 -> Add/1
  amp/1 -> MATLAB Function3/1(amp)
  Mux/1 -> Scope/1
  MATLAB Function3/2(lock_out) -> Scope9/1
  MATLAB Function3/3(c_out) -> Contador de Ciclos/1
  [rpm] -> Zero-Order Hold1/1
  1-D Lookup Table/1 -> Out2/1, Divide/1
  Constant8/1 -> MATLAB Function3/5(ret_max)
  MATLAB Function2/1(y) -> [Ciclos]
  Zero-Order Hold1/1 -> Lowpass Filter/1
  Constant10/1 -> MATLAB Function3/6(ret_min)
  MATLAB Function3/1(retard) -> Retardo atual/1, Add/2, 1-D Lookup Table/1
  [Ciclos] -> XY Graph1/1
  Divide/1 -> Mux/2, XY Graph1/3
  Constant2/1 -> Divide/2

== system teste_motor_v10/Motor de Sem Controle/Subsystem/Filtro ==
  Pressão com Knock : Inport
  Bandpass Filter : Subsystem  DialogController=fdesignblkfcn  InitFcn=fdesignblkfcn(gcbh, {'InitFcn'});  mask(Bandpass Filter){}
      mask help: Design a bandpass filter
      settings: CopyFcn=fdesignblkfcn(gcbh, {'CopyFcn'});
      mask Help: helpview(mapfilelocation('dsp'), 'dspbandpassfilter');
      mask Display: disp('Bandpass');
  Product2 : Product
  Scope : Scope
      settings: ActiveDisplayYMinimum=-30.943664586414695  ActiveDisplayYMaximum=278.49298127773233
  Spectrum Analyzer : SpectrumAnalyzer  Commented=on  WindowPosition=[1 1 2560 1003]  SampleRateSource=Property  SampleRate=44.1e3  PlotAsTwoSidedSpectrum=off  FrequencyScale=Log  FrequencySpan=Start and stop frequencies  StartFrequency=20  StopFrequency=20e3  AveragingMethod=Exponential  YLimits=[-4203.0621534311576397,-2203.0621534311580945]  AllowFFTLengthLessThanSamplesPerUpdate=on
  Square : Math  Operator=square
  Square Root : Sqrt
  Step1 : Step  Time=0.02  SampleTime=0
  Zero-Order Hold : ZeroOrderHold  Commented=on  SampleTime=1/1000
  Sinal filtrado : Outport
  Filtro : Outport  Port=2
  wires:
  Product2/1 -> Filtro/1, Square/1
  Pressão com Knock/1 -> Zero-Order Hold/1, Bandpass Filter/1(In)
  Bandpass Filter/1(Out) -> Product2/1
  Zero-Order Hold/1 -> Spectrum Analyzer/1
  Step1/1 -> Product2/2
  Square/1 -> Square Root/1
  Square Root/1 -> Scope/1, Sinal filtrado/1

== system teste_motor_v10/Motor de Sem Controle/Subsystem/Leituras ==
  Janela : Subsystem
  Knock : Subsystem
  PS-Simulink Converter : nesl_utility/PS-Simulink Converter  PhysicalDomain=network_engine_domain  SubClassName=ps_output  LeftPortType=input  RightPortType=output  PseudoPeriodic=off  Frequencies=[]  VectorFormat=inherit  Unit=inherit  AffineConversion=off
  PS-Simulink Converter1 : nesl_utility/PS-Simulink Converter  PhysicalDomain=network_engine_domain  SubClassName=ps_output  LeftPortType=input  RightPortType=output  PseudoPeriodic=off  Frequencies=[]  VectorFormat=inherit  Unit=kPa  AffineConversion=off
  Sum : Sum  Inputs=++|
  To Workspace : ToWorkspace  VariableName=ang  SaveFormat=Timeseries  SampleTime=-1
  To Workspace1 : ToWorkspace  VariableName=pressao  SaveFormat=Timeseries  SampleTime=-1
  XY Graph : Record  NumPorts=2.0  FileSettingsInternal="{\"entries\":[{\"content\":{\"excelSettings\":{\"content\":{},\"type\":\"Streamout.ExcelSettings\"},\"parquetSettings\":{\"content\":{},\"type\":\"Streamout.ParquetSettings\"}},\"type\":\"Streamout.FileSettingStorage\",\"uuid\":\"\"}],\"packageUris\":[\"http:\\/\\/schema.mathworks.com\\/mf0\\/streamout_blocks\\/R2020a\"],\"version\":\"1.0\"}"  FrameSettings=[0, 0]  Layout=[1 1]  SignalsInternal="{\"entries\":[{\"content\":{\"signals\":[{\"content\":{\"blockPath\":[],\"dimensions\":[1],\"domain\":\"\",\"lineColor\":\"#edb120\",\"lineWidth\":2,\"port\":1,\"sid\":[\"\"],\"signalID\":1,\"signalName\":\"PS-Simulink\\nConverter\"},\"type\":\"RecordBlkView.Signal\",\"uuid\":\"\"},{\"content\":{\"blockPath\":[],\"dimensions\":[1],\"domain\":\"\",\"lineColor\":\"#7e2f8e\",\"lineWidth\":2,\"port\":2,\"sid\":[\"\"],\"signalID\":2,\"signalName\":\"Sum\"},\"type\":\"RecordBlkView.Signal\",\"uuid\":\"\"}]},\"type\":\"RecordBlkView.InputSignals\",\"uuid\":\"\"}],\"packageUris\":[\"http:\\/\\/schema.mathworks.com\\/mf0\\/streamout_blocks\\/R2020a\"],\"version\":\"1.0\"}"  VisualizationBindings="{\"sparklinesplugin\":{\"info\":[{\"bindingParametersList\":[],\"subplotID\":1}]}}"  CompatibilityTag=XY
  Crank Angle : PMIOPort  Side=Left
  Pressão : PMIOPort  Port=2  Side=Left
  Pressão com Knock : Outport
  CrkAng : Outport  Port=2
  wires:
  PS-Simulink Converter/1 -> Janela/1(In1), CrkAng/1, To Workspace/1, XY Graph/1
  PS-Simulink Converter1/1 -> Sum/2
  Sum/1 -> To Workspace1/1, Pressão com Knock/1, XY Graph/2
  Janela/1(Out1) -> Knock/1(In1)
  Knock/1(Out1) -> Sum/1
  connections:
  Crank Angle/RConn1 -- PS-Simulink Converter/LConn1
  PS-Simulink Converter1/LConn1 -- Pressão/RConn1

== system teste_motor_v10/Motor de Sem Controle/Subsystem/Threshold e Sensor ==
  Sinal filtrado : Inport
  Detect Rise Positive1 : simulink/Logic and Bit Operations/Detect Rise Positive  vinit=0  OutDataTypeStr=boolean
  Product : Product
  Threshold : simulink/Logic and Bit Operations/Compare To Constant  relop=>  const=240  OutDataTypeStr=boolean
  Knock : Outport
  Amplitude : Outport  Port=2
  wires:
  Sinal filtrado/1 -> Product/2, Threshold/1
  Threshold/1 -> Detect Rise Positive1/1
  Detect Rise Positive1/1 -> Knock/1, Product/1
  Product/1 -> Amplitude/1

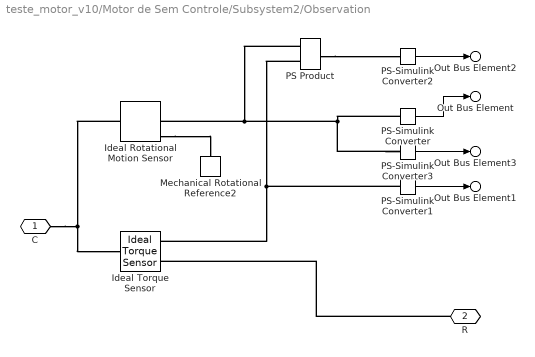
== system teste_motor_v10/Motor de Sem Controle/Subsystem2/Observation ==
  Ideal Rotational Motion Sensor : fl_lib/Mechanical/Mechanical Sensors/Ideal Rotational Motion Sensor  reference=foundation.enum.MeasurementReference.difference  acceleration_port=false  velocity_port=true  position_port=true  wrap_angle=simscape.enum.onoff.off  offset=0 rad
  Ideal Torque Sensor : fl_lib/Mechanical/Mechanical Sensors/Ideal Torque Sensor
  Mechanical Rotational Reference2 : fl_lib/Mechanical/Rotational Elements/Mechanical Rotational Reference
  PS Product : fl_lib/Physical Signals/Functions/PS Product
  PS-Simulink Converter : nesl_utility/PS-Simulink Converter  PhysicalDomain=network_engine_domain  SubClassName=ps_output  LeftPortType=input  RightPortType=output  PseudoPeriodic=off  Frequencies=[]  VectorFormat=inherit  Unit=rpm  AffineConversion=off
  PS-Simulink Converter1 : nesl_utility/PS-Simulink Converter  PhysicalDomain=network_engine_domain  SubClassName=ps_output  LeftPortType=input  RightPortType=output  PseudoPeriodic=off  Frequencies=[]  VectorFormat=inherit  Unit=N*m  AffineConversion=off
  PS-Simulink Converter2 : nesl_utility/PS-Simulink Converter  PhysicalDomain=network_engine_domain  SubClassName=ps_output  LeftPortType=input  RightPortType=output  PseudoPeriodic=off  Frequencies=[]  VectorFormat=inherit  Unit=kW  AffineConversion=off
  PS-Simulink Converter3 : nesl_utility/PS-Simulink Converter  PhysicalDomain=network_engine_domain  SubClassName=ps_output  LeftPortType=input  RightPortType=output  PseudoPeriodic=off  Frequencies=[]  VectorFormat=inherit  Unit=rad/s  AffineConversion=off
  C : PMIOPort  Side=Left
  R : PMIOPort  Port=2  Side=Right
  Out Bus Element : Outport  PortName=Info  Element=EngineSpeed
      settings: AttributesFormatString=%<Unit>
  Out Bus Element1 : Outport  PortName=Info  Element=BrakeTorque
      settings: AttributesFormatString=%<Unit>
  Out Bus Element2 : Outport  PortName=Info  Element=BrakePower
      settings: AttributesFormatString=%<Unit>
  Out Bus Element3 : Outport  PortName=Info  Element=EngineAngVel
      settings: AttributesFormatString=%<Unit>
  wires:
  PS-Simulink Converter/1 -> Out Bus Element/1
  PS-Simulink Converter1/1 -> Out Bus Element1/1
  PS-Simulink Converter2/1 -> Out Bus Element2/1
  PS-Simulink Converter3/1 -> Out Bus Element3/1
  connections:
  Ideal Rotational Motion Sensor/RConn1 -- Mechanical Rotational Reference2/LConn1
  Ideal Rotational Motion Sensor/LConn1 -- C/RConn1 -- Ideal Torque Sensor/LConn1
  PS-Simulink Converter/LConn1 -- PS-Simulink Converter3/LConn1 -- PS Product/LConn1 -- Ideal Rotational Motion Sensor/RConn2
  PS-Simulink Converter1/LConn1 -- PS Product/LConn2 -- Ideal Torque Sensor/RConn2
  R/RConn1 -- Ideal Torque Sensor/RConn1
  PS Product/RConn1 -- PS-Simulink Converter2/LConn1

== system teste_motor_v10/Motor de Sem Controle/Subsystem2/Subsystem1 ==
  Medições : Subsystem
  Scope : Scope  Commented=on  NumInputPorts=3
      settings: ActiveDisplayYMinimum=-1  ActiveDisplayYMaximum=1
  Conn1 : PMIOPort  Side=Left
  Conn2 : PMIOPort  Port=2  Side=Right
  Conn3 : PMIOPort  Port=3  Side=Right
  POS : Outport
  wires:
  Medições/3(Pressão) -> Scope/3
  Medições/2(Filtro1) -> Scope/2
  Medições/1(Grandeza) -> Scope/1
  Medições/4(POS) -> POS/1
  connections:
  Medições/RConn2 -- Conn3/RConn1
  Medições/RConn1 -- Conn2/RConn1
  Medições/LConn1 -- Conn1/RConn1

== system teste_motor_v10/Motor de com Controle/Medições/CrkAng ==
  <EngineAngVel> : Inport
  Constant : Constant  Value=720
  Gain : Gain  Gain=180/pi
  Integrator : Integrator
  Mod : Math  Operator=mod
  CrkAng : Outport
  wires:
  Gain/1 -> Mod/1
  Integrator/1 -> Gain/1
  <EngineAngVel>/1 -> Integrator/1
  Mod/1 -> CrkAng/1
  Constant/1 -> Mod/2

== system teste_motor_v10/Motor de com Controle/Medições/Filtro ==
  In1 : Inport
  Bandpass Filter : Subsystem  DialogController=fdesignblkfcn  InitFcn=fdesignblkfcn(gcbh, {'InitFcn'});  mask(Bandpass Filter){}
      mask help: Design a bandpass filter
      settings: CopyFcn=fdesignblkfcn(gcbh, {'CopyFcn'});
      mask Help: helpview(mapfilelocation('dsp'), 'dspbandpassfilter');
      mask Display: disp('Bandpass');
  Product : Product
  Product1 : Product
  Repeating Sequence : simulink/Sources/Repeating Sequence  rep_seq_t=[0, 10]  rep_seq_y=[1, 1]
  Scope : Scope  NumInputPorts=2
      settings: ActiveDisplayYMinimum=-3429.31303  ActiveDisplayYMaximum=3539.49904  DataLoggingVariableName=ScopeData4
  Step1 : Step  Time=8  SampleTime=0
  Subsystem1 : Subsystem
  Subsystem2 : Subsystem
  Sum : Sum
  Filtro : Outport
  Pressão : Outport  Port=2
  wires:
  Bandpass Filter/1(Out) -> Scope/2, Product1/1
  Sum/1 -> Pressão/1, Bandpass Filter/1(In)
  [rpm1] -> Subsystem1/1(RPM)
  Step1/1 -> Product1/2
  Product1/1 -> Filtro/1
  In1/1 -> Sum/1
  Subsystem2/1(Output) -> Product/2
  Repeating Sequence/1 -> Product/1
  [rpm1] -> Subsystem2/1(RPM)
  Product/1 -> Scope/1, Sum/2

== system teste_motor_v10/Motor de com Controle/Medições/Leitura de pressão ==
  Absolute Reference (G) : fl_lib/Gas/Elements/Absolute Reference (G)
      settings: InternalSimscapePortConfiguration="{\"Bottom\":[],\"Left\":[{\"id\":\"A\",\"label\":\"\",\"type\":\"foundation.gas.gas\"}],\"Right\":[],\"Top\":[]}"
  Load Inertia : fl_lib/Mechanical/Rotational Elements/Inertia  inertia=10*0.1^2 kg*m^2  num_ports=foundation.enum.numPorts2.one  w_specify=on  w_priority=None  w=0 rpm  w_nominal_specify=off  w_nominal_value=1  w_nominal_unit=rad/s  t_specify=off  t_priority=None  t=0 N*m  t_nominal_specify=off  t_nominal_value=1  t_nominal_unit=N*m
      settings: AttributesFormatString=|
      | Initial: %<w> [%<w_unit>]
      | %<inertia> [%<inertia_unit>]
  PS-Simulink Converter4 : nesl_utility/PS-Simulink Converter  PhysicalDomain=network_engine_domain  SubClassName=ps_output  LeftPortType=input  RightPortType=output  PseudoPeriodic=off  Frequencies=[]  VectorFormat=inherit  Unit=Pa  AffineConversion=off
  Pressure & Temperature Sensor (G) : fl_lib/Gas/Sensors/Pressure & Temperature Sensor (G)  reference=foundation.enum.MeasurementReference.difference  pressure=true  pressure_spec=foundation.enum.PressureMeasementSpec.Absolute  temperature=true
      settings: InternalSimscapePortConfiguration="{\"Bottom\":[{\"id\":\"T\",\"label\":\"T\",\"type\":\"output\"}],\"Left\":[{\"id\":\"A\",\"label\":\"A\",\"type\":\"foundation.gas.gas\"}],\"Right\":[{\"id\":\"B\",\"label\":\"B\",\"type\":\"foundation.gas.gas\"},{\"id\":\"P\",\"label\":\"P\",\"type\":\"output\"}],\"Top\":[]}"
  Rotational Mechanical Converter (G) : fl_lib/Gas/Elements/Rotational Mechanical Converter (G)  mech_orientation=foundation.enum.MechOrientationRotational.Negative  rotation_spec=foundation.enum.RotationSpec.Calculate  theta_init=0 rad  volume_displacement=0.01 m^3/rad  dead_volume=1e-5 m^3  area_A=0.01 m^2  environment_spec=foundation.enum.pressure_spec.atmospheric  environment_pressure=0.101325 MPa  p_I_specify=off  p_I_priority=High  p_I=0.101325 MPa  p_I_nominal_specify=off  p_I_nominal_value=1  p_I_nominal_unit=MPa  T_I_specify=off  T_I_priority=High  T_I=293.15 K  T_I_nominal_specify=off  T_I_nominal_value=1  T_I_nominal_unit=K  rho_I_specify=off  rho_I_priority=High  rho_I=0.715 kg/m^3  rho_I_nominal_specify=off  rho_I_nominal_value=1  rho_I_nominal_unit=kg/m^3
      settings: InternalSimscapePortConfiguration="{\"Bottom\":[],\"Left\":[{\"id\":\"A\",\"label\":\"A\",\"type\":\"foundation.gas.gas\"},{\"id\":\"R\",\"label\":\"R\",\"type\":\"foundation.mechanical.rotational.rotational\"}],\"Right\":[{\"id\":\"H\",\"label\":\"H\",\"type\":\"foundation.thermal.thermal\"},{\"id\":\"C\",\"label\":\"C\",\"type\":\"foundation.mechanical.rotational.rotational\"}],\"Top\":[]}"
  Conn1 : PMIOPort  Side=Left
  Conn2 : PMIOPort  Port=2  Side=Right
  Conn3 : PMIOPort  Port=3  Side=Right
  output : Outport
  wires:
  PS-Simulink Converter4/1 -> output/1
  connections:
  Pressure & Temperature Sensor (G)/RConn3 -- Conn2/RConn1
  Rotational Mechanical Converter (G)/LConn1 -- Pressure & Temperature Sensor (G)/LConn1
  Load Inertia/LConn1 -- Rotational Mechanical Converter (G)/RConn2
  Pressure & Temperature Sensor (G)/RConn2 -- PS-Simulink Converter4/LConn1
  Rotational Mechanical Converter (G)/RConn1 -- Conn3/RConn1
  Pressure & Temperature Sensor (G)/RConn1 -- Absolute Reference (G)/LConn1
  Rotational Mechanical Converter (G)/LConn2 -- Conn1/RConn1

== system teste_motor_v10/Motor de com Controle/Medições/Sensor ==
  CrkAng : Inport
  Filtro : Inport  Port=2
  Product : Product
  Sensor : Subsystem
  Square : Math  Operator=square
  Square Root : Sqrt
  Subsystem4 : Subsystem
  Zero-Order Hold : ZeroOrderHold  SampleTime=-1
  Grandeza : Outport
  wires:
  Zero-Order Hold/1 -> Subsystem4/1(u)
  Sensor/1(Output) -> Zero-Order Hold/1
  CrkAng/1 -> Sensor/1(In1)
  Filtro/1 -> Sensor/2(In2), Product/2
  Square Root/1 -> Grandeza/1
  Product/1 -> Square/1
  Square/1 -> Square Root/1
  Subsystem4/1(Out1) -> Product/1

== system teste_motor_v10/Motor de Sem Controle/Subsystem/Filtro/Bandpass Filter ==
  In : Inport
  Generated Filter Block : dsparch4/Biquad Filter  Tag=BlockMethodSubSystem  FilterSource=Dialog parameters  CoeffSource=Specify via dialog  FilterObject=BQF  IIRFiltStruct=Direct form II  BiQuadCoeffs=[0.546964581851781317 0 -0.546964581851781317 1 0.212586114403401139 0.068742568417802366]  ScaleValues=[0.851295917945335656;1]  IC=0  ICnum=0  ICden=0  a0Flag=Warning  optimizeScaleValues=off  ScaleValueMode=Specify via input port (g)  InputProcessing=Columns as channels (frame based)  roundingMode=Floor  overflowMode=off  scaleValueFracLength=14  denProdOutputFracLength=30  denAccumFracLength=30  secondMemoryFracLength=15
  Out : Outport  VectorParamsAs1DForOutWhenUnconnected=off
  wires:
  In/1 -> Generated Filter Block/1
  Generated Filter Block/1 -> Out/1
